simulink model "DCDC_ClosedLoop1"  (R2023b)
settings: Solver=ode23tb  StartTime=0.0  StopTime=0.2  MaxStep=1e-5  RelTol=1e-3  AbsTol=1e-3
InitFcn:
  | init_DCDC_ClosedLoop;
StopFcn:
  | PlotResults;
values from neighbouring files (symbols this model uses):
  Co = DCDC_Co*(10^-6)    [init_DCDC_ClosedLoop.m]
  I_load = Pout/DCDC_vout    [DC_DC_Converter.m]    (also in Data_DCDC_converter.mat = 212.5)
  IinMax = I_in_rated    [init_DCDC_ClosedLoop.m]
  Iload = I_load    [init_DCDC_ClosedLoop.m]
  kii = wzi *kpi    [DC_DC_Converter.m]    (also in Data_DCDC_converter.mat = 2106.71507358; init_DCDC_ClosedLoop.m = wzi*kpi)
  kiv = kpv*wzv    [DC_DC_Converter.m]    (also in Data_DCDC_converter.mat = 443.093490604; init_DCDC_ClosedLoop.m)
  kpi = L*wc_i    [DC_DC_Converter.m]    (also in Data_DCDC_converter.mat = 1.75559589465; init_DCDC_ClosedLoop.m = wci*Lin)
  kpv = (DCDC_Co*10^-6)*wc_v    [DC_DC_Converter.m]    (also in Data_DCDC_converter.mat = 0.678584013175; init_DCDC_ClosedLoop.m = wcv*Co)
  Lin = L    [init_DCDC_ClosedLoop.m]
  Tau_d = 1.5*Ts    [init_DCDC_ClosedLoop.m]
  TimeEnable = 5e-3    (= 0.005)    [init_DCDC_ClosedLoop.m]
  TimeLoad = 0.06    [init_DCDC_ClosedLoop.m]
  Trise = 25e-3    (= 0.025)    [init_DCDC_ClosedLoop.m]
  Ts = 1/fs    [init_DCDC_ClosedLoop.m]
  Vbat = DCDC_vbatt    [init_DCDC_ClosedLoop.m]
  VdcSetpoint = DCDC_vout    [init_DCDC_ClosedLoop.m]
libraries: simulink x2
settings Model: Creator=radubojoi  LastModifiedBy=giuse
settings RTWCC: GPUComputeCapability=5.0

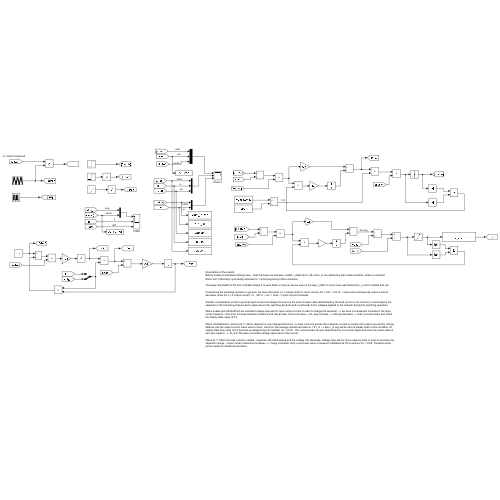
[thumbnail: Simulink's stored preview of the top-level diagram]
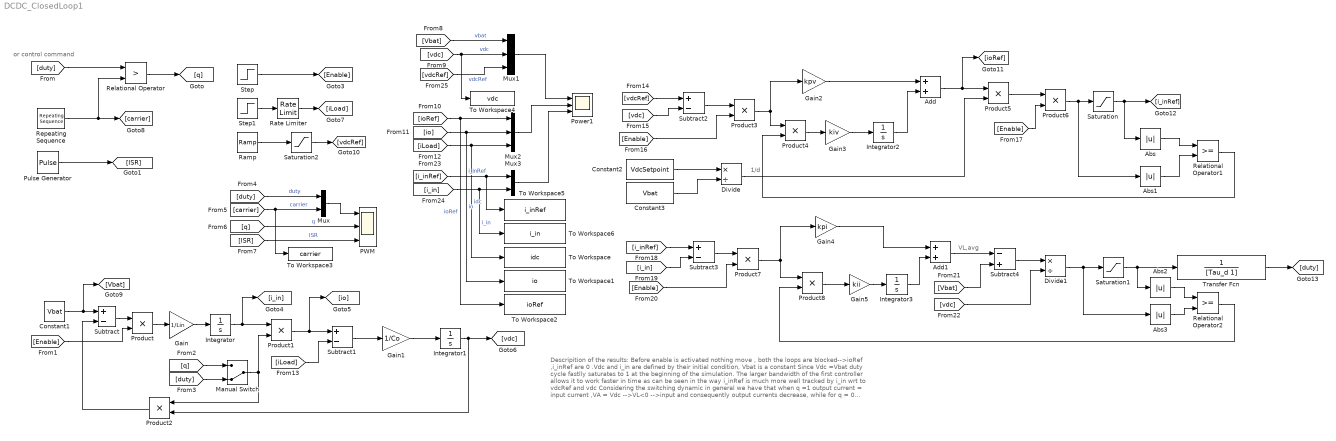
== system DCDC_ClosedLoop1 ==
  note: 1/d
  note: or control command
  note: VL,avg
  note: Descripition of the results:
      | Before enable is activated nothing move , both the loops are blocked-->ioRef ,i_inRef are 0 .Vdc and i_in are defined by their initial condition, Vbat is a constant
      | Since Vdc =Vbat duty cycle fastlly saturates to 1 at the beginning of the simulation.
      |
      | The larger bandwidth of the first controller allows it to work faster in time as can be seen in the way i_inRef is much more well tracked by i_in wrt to vdcRef and vdc
      |
      | Considering the switching dynamic in general  we have that when q =1 output current = input current ,VA = Vdc -->VL<0 -->input and consequently output currents decrease, while for q = 0 output current = 0 , VA= 0 -->VL = Vbat --> input current increases.
      |
      | Another consideration is that in general input current can always be seen as the sum of mean value determined by the load current or dc current (or eventually by the capacitor in the transitory phases) and a ripple due to the switching dynamic and in particular to the voltages applied to the inductor during the switching operation
      |
      | When enable and VdcSetPoint are activated voltage loop ask for more output current in order to charge the capacitor --> we have a consequent increase in the input current request -->the error increase between reference and actual input current increase -->VL,avg increase ---->VA,avg decrease --> duty cycle decrease and reach the steady state value of 0.5
      |
      | When VdcSetPoint is reached at t = 30ms capacitor is now charged and since  no load current is present the capacitor current is equal to the output one and for charge balance rule the output current mean value is zero.  Since for the average dynamical model io = d*i_in --> also i_in,avg will be zero at steady state in this condition. At steady state duty cycle is 0.5 because we always have to maintain Vo = Vin/d . The current peaks are just determined by the current ripple and since the mean value is zero are equal to   +- dI_in/2. We have just a little voltage ripple due to this current.
      |
      | When at t = 60ms the load current is added , capacitor start discharging and the voltage Vdc decrease. Voltage loop ask for more output current in order to maintain the capacitor charge -->input current reference increases --> VLavg increases .Duty cycle mean value is however maintaned at 0.5 to ensure Vo = Vin/d. Therefore input current ripple is maintaned as before.
      |
      | When at t = 110ms the load current reach is maximum value, input current oscillates instantaneously around the mean rated value of 425A (considering the converter ideal since we are talking about a model) and with a the same always ripple determined by the same duty cycle.
  Abs{,1..3} (4 alike) : Abs  SaturateOnIntegerOverflow=off
  Add : Sum
  Add1 : Sum
  Constant1 : Constant  Value=Vbat
  Constant2 : Constant  Value=VdcSetpoint
  Constant3 : Constant  Value=Vbat
  Divide : Product  Inputs=*/
  Divide1 : Product  Inputs=*/
  Gain : Gain  Gain=1/Lin
  Gain1 : Gain  Gain=1/Co
  Gain2 : Gain  Gain=kpv
  Gain3 : Gain  Gain=kiv
  Gain4 : Gain  Gain=kpi
  Gain5 : Gain  Gain=kii
  Integrator : Integrator
  Integrator1 : Integrator  InitialCondition=Vbat
  Integrator2 : Integrator
  Integrator3 : Integrator
  Manual Switch : ManualSwitch  CurrentSetting=0
  Mux : Mux  Inputs=2
  Mux1 : Mux  Inputs=3
  Mux2 : Mux  Inputs=3
  Mux3 : Mux  Inputs=2
  PWM : Scope  NumInputPorts=3
  Power1 : Scope  NumInputPorts=3
  Product{,1..8} (9 alike) : Product
  Pulse Generator : DiscretePulseGenerator  PulseType=Time based  Period=Ts  PulseWidth=50
  Ramp : simulink/Sources/Ramp  slope=(VdcSetpoint-Vbat)/Trise  start=TimeEnable  InitialOutput=Vbat
  Rate Limiter : RateLimiter  RisingSlewLimit=I_load/50e-3  FallingSlewLimit=-I_load/50e-3  SampleTimeMode=inherited
  Relational Operator : RelationalOperator  Operator=>  RndMeth=Simplest  InputSameDT=off
  Relational Operator1 : RelationalOperator  RndMeth=Simplest
  Relational Operator2 : RelationalOperator  RndMeth=Simplest
  Repeating Sequence : simulink/Sources/Repeating Sequence  rep_seq_t=[0 Ts/2 Ts]  rep_seq_y=[0 1 0]
  Saturation : Saturate  UpperLimit=IinMax  LowerLimit=-IinMax
  Saturation1 : Saturate  UpperLimit=1  LowerLimit=0.1
  Saturation2 : Saturate  UpperLimit=VdcSetpoint  LowerLimit=Vbat
  Step : Step  Time=TimeEnable  SampleTime=0
  Step1 : Step  Time=TimeLoad  After=Iload  SampleTime=0
  Subtract{,1..3} (4 alike) : Sum  Inputs=+-
  Subtract4 : Sum  Inputs=-+
  To Workspace : ToWorkspace  VariableName=idc  SampleTime=-1
  To Workspace1 : ToWorkspace  VariableName=io  SampleTime=-1
  To Workspace2 : ToWorkspace  VariableName=ioRef  SampleTime=-1
  To Workspace3 : ToWorkspace  VariableName=carrier  SampleTime=-1
  To Workspace4 : ToWorkspace  VariableName=vdc  SampleTime=-1
  To Workspace5 : ToWorkspace  VariableName=i_inRef  SampleTime=-1
  To Workspace6 : ToWorkspace  VariableName=i_in  SampleTime=-1
  Transfer Fcn : TransferFcn  Denominator=[Tau_d 1]
  wires:
  Repeating Sequence/1 -> [carrier], Relational Operator/2
  [duty] -> Relational Operator/1
  Relational Operator/1 -> [q]
  Pulse Generator/1 -> [ISR]
  Step/1 -> [Enable]
  Constant1/1 -> [Vbat], Subtract/1
  Subtract/1 -> Product/1
  [Enable] -> Product/2
  Product/1 -> Gain/1
  Gain/1 -> Integrator/1
  [q] -> Manual Switch/1
  [duty] -> Manual Switch/2
  Integrator/1 -> Product1/1, [i_in]
  Manual Switch/1 -> Product2/1, Product1/2
  Product2/1 -> Subtract/2
  Product1/1 -> [io], Subtract1/1
  Subtract1/1 -> Gain1/1
  Gain1/1 -> Integrator1/1
  Integrator1/1 -> [vdc], Product2/2
  [duty] -> Mux/1  "duty"
  [carrier] -> To Workspace3/1, Mux/2  "carrier"
  Mux/1 -> PWM/1
  [q] -> PWM/2  "q"
  [ISR] -> PWM/3  "ISR"
  [Vbat] -> Mux1/1  "vbat"
  [vdc] -> To Workspace4/1, Mux1/2  "vdc"
  [io] -> Mux2/2, To Workspace1/1  "io"
  [ioRef] -> To Workspace2/1, Mux2/1  "ioRef"
  [iLoad] -> Mux2/3, To Workspace/1  "idc"
  Mux1/1 -> Power1/1
  Mux2/1 -> Power1/2
  [iLoad] -> Subtract1/2
  Ramp/1 -> Saturation2/1
  Saturation2/1 -> [vdcRef]
  [vdcRef] -> Subtract2/1
  [vdc] -> Subtract2/2
  Subtract2/1 -> Product3/1
  [Enable] -> Product3/2
  Product4/1 -> Gain3/1
  Product3/1 -> Product4/1, Gain2/1
  Gain3/1 -> Integrator2/1
  Gain2/1 -> Add/1
  Integrator2/1 -> Add/2
  Add/1 -> [ioRef], Product5/1
  Product5/1 -> Product6/1
  [Enable] -> Product6/2
  Constant2/1 -> Divide/1
  Constant3/1 -> Divide/2
  Divide/1 -> Product5/2
  Product6/1 -> Abs1/1, Saturation/1
  Saturation/1 -> Abs/1, [i_inRef]
  Abs/1 -> Relational Operator1/1
  Abs1/1 -> Relational Operator1/2
  Relational Operator1/1 -> Product4/2
  [i_inRef] -> Subtract3/1
  [i_in] -> Subtract3/2
  Subtract3/1 -> Product7/1
  [Enable] -> Product7/2
  Product7/1 -> Product8/1, Gain4/1
  Gain5/1 -> Integrator3/1
  Gain4/1 -> Add1/1
  Integrator3/1 -> Add1/2
  Product8/1 -> Gain5/1
  Add1/1 -> Subtract4/1
  [Vbat] -> Subtract4/2
  Subtract4/1 -> Divide1/1
  [vdc] -> Divide1/2
  Divide1/1 -> Abs3/1, Saturation1/1
  Saturation1/1 -> Transfer Fcn/1, Abs2/1
  Abs2/1 -> Relational Operator2/1
  Abs3/1 -> Relational Operator2/2
  Relational Operator2/1 -> Product8/2
  Transfer Fcn/1 -> [duty]
  [i_inRef] -> To Workspace5/1, Mux3/1  "i_inRef"
  [i_in] -> To Workspace6/1, Mux3/2  "i_in"
  Mux3/1 -> Power1/3
  [vdcRef] -> Mux1/3  "vdcRef"
  Step1/1 -> Rate Limiter/1
  Rate Limiter/1 -> [iLoad]
